simulink model "MySimulationModel"  (R2024b)
settings: Solver=VariableStepAuto  StartTime=0.0  StopTime=10.0  RelTol=1e-3
settings Model: Creator=xinxing  LastModifiedBy=xinxing

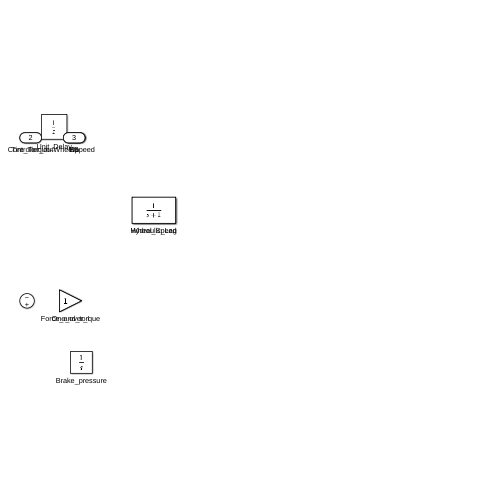
[thumbnail: Simulink's stored preview of the top-level diagram]
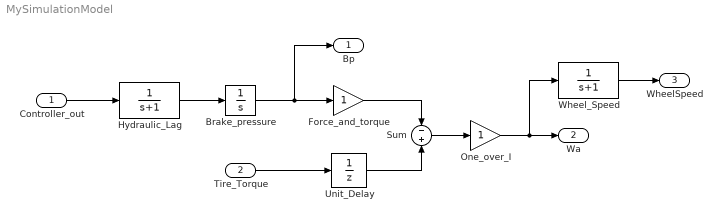
== system MySimulationModel ==
  Controller_out : Inport
  Tire_Torque : Inport  Port=2
  Brake_pressure : Integrator
  Force_and_torque : Gain
  Hydraulic_Lag : TransferFcn  Denominator=[1 1]
  One_over_I : Gain
  Sum : Sum  Inputs=-+
  Unit_Delay : UnitDelay  SampleTime=-1  HasFrameUpgradeWarning=on
  Wheel_Speed : TransferFcn  Denominator=[1 1]
  Bp : Outport
  Wa : Outport  Port=2
  WheelSpeed : Outport  Port=3
  wires:
  Wheel_Speed/1 -> WheelSpeed/1
  Unit_Delay/1 -> Sum/2
  Force_and_torque/1 -> Sum/1
  Tire_Torque/1 -> Unit_Delay/1
  Sum/1 -> One_over_I/1
  Brake_pressure/1 -> Bp/1, Force_and_torque/1
  Hydraulic_Lag/1 -> Brake_pressure/1
  One_over_I/1 -> Wa/1, Wheel_Speed/1
  Controller_out/1 -> Hydraulic_Lag/1
